simulink model "HybridControllerD2D2"  (R2019a)
settings: Solver=FixedStepDiscrete  StartTime=0.0  StopTime=inf  FixedStep=samplePeriod  RelTol=1e-3  AbsTol=1e-6  EnableMultiTasking=on
PreLoadFcn:
  | initializeSimulation;
  | ATS_setup;
InitFcn:
  | clear('all');
  | initializeSimulation;
  | ATS_setup;
values from neighbouring files (symbols this model uses):
  damperA = 0    [initializeSimulation.m]
  damperB = 0    [initializeSimulation.m]
  damperC = 0    [initializeSimulation.m]
  damperCanon = 1    [initializeSimulation.m]
  flowCanon = 3.85    [initializeSimulation.m]
  forceCanon = 1    [initializeSimulation.m]
  frictionA = 0    [initializeSimulation.m]
  frictionB = 0    [initializeSimulation.m]
  frictionC = 0    [initializeSimulation.m]
  gasConstant = 1.8    [initializeSimulation.m]
  lengthCanon = 1    [initializeSimulation.m]
  massA = 4.2    [initializeSimulation.m]
  massB = 2.5    [initializeSimulation.m]
  massC = 2.5    [initializeSimulation.m]
  massCanon = 0.002588    [initializeSimulation.m]
  maxDisplA = (stroke2A + endLength2A) * lengthCanon    (= 22)    [initializeSimulation.m]
  maxDisplB = (stroke2B + endLength2B) * lengthCanon    (= 42)    [initializeSimulation.m]
  maxDisplC = (stroke2C + endLength2C) * lengthCanon    (= 72)    [initializeSimulation.m]
  maxOilVolume = volume * (1 - (precharge/supplyPress)^(1/gasConstant))    (= 10.5071802963)    [initializeSimulation.m]
  maxVelocA = (maxFlowA * flowCanon / (area1A * areaCanon)) / velocCanon    [initializeSimulation.m]
  maxVelocB = (maxFlowB * flowCanon / (area1B * areaCanon)) / velocCanon    [initializeSimulation.m]
  maxVelocC = (maxFlowC * flowCanon / (area1C * areaCanon)) / velocCanon    [initializeSimulation.m]
  minDisplA = -(stroke1A + endLength1A) * lengthCanon    (= -22)    [initializeSimulation.m]
  minDisplB = -(stroke1B + endLength1B) * lengthCanon    (= -42)    [initializeSimulation.m]
  minDisplC = -(stroke1C + endLength1C) * lengthCanon    (= -72)    [initializeSimulation.m]
  minVelocA = -(maxFlowA * flowCanon / (area2A * areaCanon)) / velocCanon    [initializeSimulation.m]
  minVelocB = -(maxFlowB * flowCanon / (area2B * areaCanon)) / velocCanon    [initializeSimulation.m]
  minVelocC = -(maxFlowC * flowCanon / (area2C * areaCanon)) / velocCanon    [initializeSimulation.m]
  MRC = [2 0.05 0.001]    [ATS_setup.m]
  nAct = 8    [initializeSimulation.m]
  nAdcU = 12    [initializeSimulation.m]
  nDinp = 4    [initializeSimulation.m]
  nDout = 4    [initializeSimulation.m]
  nDucU = 8    [initializeSimulation.m]
  nEncU = 2    [initializeSimulation.m]
  Nl = floor(tl*sample_rate)    [ATS_setup.m]
  P_range = [0.7 1.30 ... (first row only)    [ATS_setup.m]
  precharge = 1000    [initializeSimulation.m]
  pumpFlow = 1e10    (= 10000000000)    [initializeSimulation.m]
  returnPress = 50    [initializeSimulation.m]
  SN = 16    [ATS_setup.m]
  staticForceA = 0    [initializeSimulation.m]
  staticForceB = 0    [initializeSimulation.m]
  staticForceC = 0    [initializeSimulation.m]
  supplyPress = 3000    [initializeSimulation.m]
  velocCanon = 1    [initializeSimulation.m]
  volume = accumVolume * accumNumber    (= 23)    [initializeSimulation.m]
  volumeCanon = 231    [initializeSimulation.m]
  yieldDisplA = 0.1    [initializeSimulation.m]
  yieldDisplB = 0.1    [initializeSimulation.m]
  yieldDisplC = 0.1    [initializeSimulation.m]
  Zden = ztag.Denominator{1}    [ATS_setup.m]
  Znum = ztag.Numerator{1}    [ATS_setup.m]
undefined symbols (not defined in the file or in its folder): DiscIntNeverNeededParam, HybridCtrlParameters, Par, Threshold
libraries: simulink x13
(part 1 of 3)
settings Model: ExtModeTrigMode=oneshot  ExtModeArmWhenConnect=off  ExtModeAutoUpdateStatusClock=off  Creator=Andreas Schellenberg  LastModifiedBy=Andreas
settings SolverCC: AutoScaleAbsTol=off
settings DataIOCC: SaveFormat=Array  SaveOutput=off  SaveTime=off  ReturnWorkspaceOutputs=off  SignalLoggingName=sigsOut
settings OptimizationCC: ExpressionDepthLimit=2147483647  InitFltsAndDblsToZero=on  LifeSpan=inf
settings DebuggingCC: SaveWithParameterizedLinksMsg=none  CheckSSInitialOutputMsg=off  UnderspecifiedInitializationDetection=Classic  MergeDetectMultiDrivingBlocksExec=none  MultiTaskDSMMsg=warning  MultiTaskCondExecSysMsg=none  AllowSymbolicDim=off  StateNameClashWarn=warning  SFUnexpectedBacktrackingDiag=warning  SFNoUnconditionalDefaultTransitionDiag=warning  SFExecutionAtInitializationDiag=none  ArithmeticOperatorsInVariantConditions=warning
settings HardwareCC: ProdBitPerPointer=32  ProdBitPerSizeT=32  ProdBitPerPtrDiffT=32  ProdLargestAtomicFloat=None  ProdIntDivRoundTo=Undefined  ProdEndianess=Unspecified  ProdWordSize=32  ProdHWDeviceType=32-bit Generic  TargetUnknown=on
settings ModelReferenceCC: PropagateSignalLabelsOutOfModel=off
settings SFSimCC: SimCustomHeaderCode="#include \"PredictorCorrector.h\""  SimUserSources=PredictorCorrector.c  SimUseLocalCustomCode=off  SimParseCustomCode=off
settings RTWCC: Description=Generic Real-Time Target  RTWUseLocalCustomCode=off
settings CodeAppCC: StateflowObjectComments=on
settings GRTTargetCC: TargetFcnLib=ansi_tfl_tmw.mat  TargetLangStandard=C89/C90 (ANSI)  GeneratePreprocessorConditionals=Disable all  CombineOutputUpdateFcns=off  GRTInterface=on
settings ConfigComp: CovMetricSettings=dw  CovHtmlReporting=on  CovSaveCumulativeToWorkspaceVar=on  CovSaveSingleToWorkspaceVar=on  CovExternalEMLEnable=off  CovSFcnEnable=off

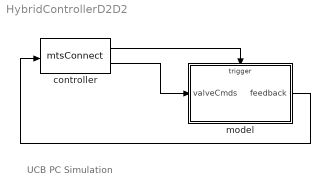
== system HybridControllerD2D2 ==
  note: UCB PC Simulation
  controller : S-Function  FunctionName=mtsConnect  Parameters='127.0.0.1',5002,nUDPInp,nUDPOut  SFunctionDeploymentMode=off  EnableBusSupport=off
  model : Subsystem  TreatAsAtomicUnit=on
  wires:
  model/1(feedback) -> controller/1
  controller/2 -> model/1(valveCmds)
  controller/1 -> model/Trigger

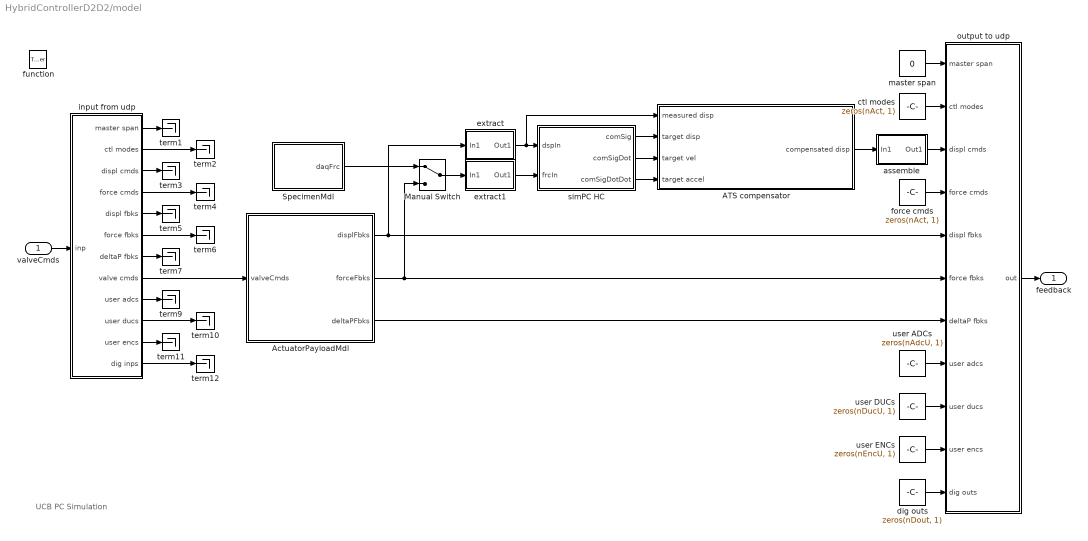
== system HybridControllerD2D2/model ==
  note: UCB PC Simulation
  valveCmds : Inport
  function : TriggerPort  TriggerType=function-call  VariantControl=(inherit)
  ATS compensator : Subsystem  mask(ATS Compensator){param=Par, threshold=Threshold}
      mask prompts: param "Initial a0, a1, a2 values :"; threshold "Threshold values :"
      mask help:
      | Adaptive Time Series (ATS) Compensator
      | by Yunbyeong Chae, Old Dominion University
      | Ref: Chae, Y., Kazemibidokhti, K., and Ricles, J.M. (2013)
      | “Adaptive time series compensator for delay compensation of servo-hydraulic actuator systems for real-time hybrid simulation”,
      | Earthquake Engineering and Structural Dynamics, 42(11), 1697-1715.
  ActuatorPayloadMdl : Subsystem
  Manual Switch : ManualSwitch
  SpecimenMdl : Subsystem
      mask Display: fprintf('Test\nSpecimen');
  assemble : Subsystem  mask(to Actuators){id=1, size=nAct}
      mask prompts: id "Index Vector: id"; size "Vector Size: size"
      mask help: To select to which actuator(s) the signals are going to
      mask Display: disp('Assemble')
  ctl modes : Constant  Value=zeros(nAct, 1)
  dig outs : Constant  Value=zeros(nDout, 1)  OutDataTypeStr=uint32
  extract : Subsystem  mask(from Actuators){id=1, size=nAct}
      mask prompts: id "Index Vector: id"; size "Vector Size: size"
      mask help: To select from which actuator(s) the signals are coming from
      mask Display: disp('Extract')
  extract1 : Subsystem  mask(from Actuators){id=1, size=nAct}
      mask prompts: id "Index Vector: id"; size "Vector Size: size"
      mask help: To select from which actuator(s) the signals are coming from
      mask Display: disp('Extract')
  force cmds : Constant  Value=zeros(nAct, 1)
  input from udp : Subsystem
  master span : Constant  Value=0
  output to udp : Subsystem
  simPC HC : Subsystem  mask(Hybrid Controller: D2/D2){nDOF=HybridCtrlParameters.nDOF, upFact=HybridCtrlParameters.upFact, dtInt=HybridCtrlParameters.dtInt, dtSim=HybridCtrlParameters.dtSim, dtCon=HybridCtrlParameters.dtCon, N=HybridCtrlParameters.N, iDelay=HybridCtrlParameters.iDelay}
      mask prompts: nDOF "Number of DOF: nDOF"; upFact "Upsample Factor: upFact"; dtInt "Integration time step: dtInt"; dtSim "Simulation time step: dtSim"; dtCon "Controller time step: dtCon"; N "Number of substeps: N"; iDelay "Number of delay steps: iDelay"
      mask help: Hybrid Controller using C0-continuous quadratic Lagrange interpolation for prediction and correction
      mask Display: disp('simPC Target\nHybrid Controller\n(D2/D2)')
  term{1..7,9..12} (11 alike) : Terminator
  user ADCs : Constant  Value=zeros(nAdcU, 1)
  user DUCs : Constant  Value=zeros(nDucU, 1)
  user ENCs : Constant  Value=zeros(nEncU, 1)
  feedback : Outport
  wires:
  input from udp/3(displ cmds) -> term3/1
  input from udp/1(master span) -> term1/1
  input from udp/6(force fbks) -> term6/1
  input from udp/10(user ducs) -> term10/1
  input from udp/12(dig inps) -> term12/1
  input from udp/2(ctl modes) -> term2/1
  input from udp/4(force cmds) -> term4/1
  input from udp/5(displ fbks) -> term5/1
  input from udp/7(deltaP fbks) -> term7/1
  input from udp/9(user adcs) -> term9/1
  input from udp/11(user encs) -> term11/1
  valveCmds/1 -> input from udp/1(inp)
  master span/1 -> output to udp/1(master span)
  ctl modes/1 -> output to udp/2(ctl modes)
  assemble/1(Out1) -> output to udp/3(displ cmds)
  force cmds/1 -> output to udp/4(force cmds)
  user ADCs/1 -> output to udp/8(user adcs)
  user DUCs/1 -> output to udp/9(user ducs)
  user ENCs/1 -> output to udp/10(user encs)
  dig outs/1 -> output to udp/11(dig outs)
  output to udp/1(out) -> feedback/1
  ActuatorPayloadMdl/1(displFbks) -> output to udp/5(displ fbks), extract/1(In1)
  ActuatorPayloadMdl/2(forceFbks) -> output to udp/6(force fbks), Manual Switch/2
  ActuatorPayloadMdl/3(deltaPFbks) -> output to udp/7(deltaP fbks)
  input from udp/8(valve cmds) -> ActuatorPayloadMdl/1(valveCmds)
  extract1/1(Out1) -> simPC HC/2(frcIn)
  extract/1(Out1) -> simPC HC/1(dspIn), ATS compensator/1(measured disp)
  simPC HC/2(comSigDot) -> ATS compensator/3(target vel)
  simPC HC/3(comSigDotDot) -> ATS compensator/4(target accel)
  ATS compensator/1(compensated disp) -> assemble/1(In1)
  simPC HC/1(comSig) -> ATS compensator/2(target disp)
  Manual Switch/1 -> extract1/1(In1)
  SpecimenMdl/1(daqFrc) -> Manual Switch/1

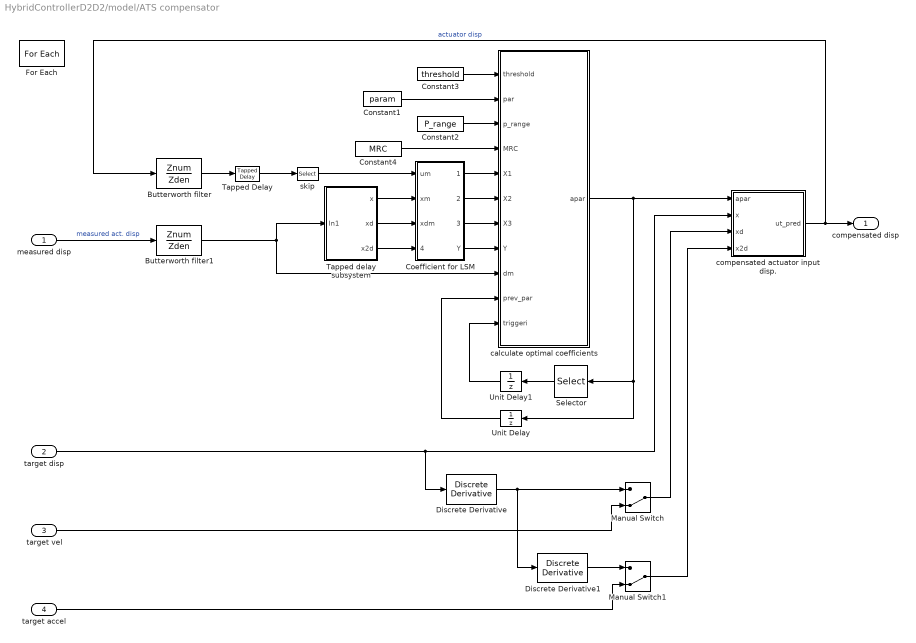
== system HybridControllerD2D2/model/ATS compensator ==
  measured disp : Inport  Partition=on  PartitionDimension=1  PartitionWidth=1  PartitionOffset=0
  target disp : Inport  Port=2  Partition=on  PartitionDimension=1  PartitionWidth=1  PartitionOffset=0
  target vel : Inport  Port=3  Partition=on  PartitionDimension=1  PartitionWidth=1  PartitionOffset=0
  target accel : Inport  Port=4  Partition=on  PartitionDimension=1  PartitionWidth=1  PartitionOffset=0
  Butterworth filter : DiscreteTransferFcn  Numerator=Znum  Denominator=Zden
  Butterworth filter1 : DiscreteTransferFcn  Numerator=Znum  Denominator=Zden
  Coefficient for LSM : Subsystem
  Constant1 : Constant  Value=param
  Constant2 : Constant  Value=P_range
  Constant3 : Constant  Value=threshold
  Constant4 : Constant  Value=MRC
  Discrete Derivative : simulink/Discrete/Discrete Derivative  gainval=1.0  ICPrevScaledInput=0.0  OutMin=[]  OutMax=[]  OutDataType=fixdt(1, 16)  OutScaling=2^-10  DoSatur=off
  Discrete Derivative1 : simulink/Discrete/Discrete Derivative  gainval=1.0  ICPrevScaledInput=0.0  OutMin=[]  OutMax=[]  OutDataType=fixdt(1, 16)  OutScaling=2^-10  DoSatur=off
  For Each : ForEach  DisableCoverage=on  IterateSubsysMaskParameter=on,on  SubsysMaskParameterIterationDimension=2,2  IndexMode=One-based
  Manual Switch : ManualSwitch  CurrentSetting=0
  Manual Switch1 : ManualSwitch  CurrentSetting=0
  Selector : Selector  InputPortWidth=4  IndexOptions=Index vector (dialog)  Indices=4  OutputSizes=1
  Tapped Delay : simulink/Discrete/Tapped Delay  vinit=0.0  samptime=-1  NumDelays=Nl  DelayOrder=Oldest  includeCurrent=off
  Tapped delay subsystem : Subsystem
  Unit Delay : UnitDelay  SampleTime=-1  HasFrameUpgradeWarning=on
  Unit Delay1 : UnitDelay  SampleTime=-1  HasFrameUpgradeWarning=on
  calculate optimal coefficients : MATLAB Function  TreatAsAtomicUnit=on
  compensated actuator input disp. : MATLAB Function  TreatAsAtomicUnit=on
  skip : Selector  InputPortWidth=Nl  IndexOptions=Index vector (dialog)  Indices=[1:SN:Nl]  OutputSizes=1
  compensated disp : Outport  ConcatenationDimension=1
  wires:
  measured disp/1 -> Butterworth filter1/1  "measured act. disp"
  Tapped Delay/1 -> skip/1
  calculate optimal coefficients/1(apar) -> Unit Delay/1, Selector/1, compensated actuator input disp./1(apar)
  compensated actuator input disp./1(ut_pred) -> Butterworth filter/1, compensated disp/1  "actuator disp"
  Constant1/1 -> calculate optimal coefficients/2(par)
  Constant2/1 -> calculate optimal coefficients/3(p_range)
  Unit Delay/1 -> calculate optimal coefficients/10(prev_par)
  target disp/1 -> compensated actuator input disp./2(x), Discrete Derivative/1
  skip/1 -> Coefficient for LSM/1(um)
  Tapped delay subsystem/1(x) -> Coefficient for LSM/2(xm)
  Tapped delay subsystem/2(xd) -> Coefficient for LSM/3(xdm)
  Tapped delay subsystem/3(x2d) -> Coefficient for LSM/4(x2dm)
  Coefficient for LSM/1(X(1,:)) -> calculate optimal coefficients/5(X1)
  Coefficient for LSM/2(X(2,:)) -> calculate optimal coefficients/6(X2)
  Coefficient for LSM/3(X(3,:)) -> calculate optimal coefficients/7(X3)
  Coefficient for LSM/4(Y) -> calculate optimal coefficients/8(Y)
  Unit Delay1/1 -> calculate optimal coefficients/11(triggeri)
  Constant3/1 -> calculate optimal coefficients/1(threshold)
  Butterworth filter/1 -> Tapped Delay/1
  Constant4/1 -> calculate optimal coefficients/4(MRC)
  Selector/1 -> Unit Delay1/1
  Manual Switch/1 -> compensated actuator input disp./3(xd)
  Discrete Derivative/1 -> Manual Switch/1, Discrete Derivative1/1
  target vel/1 -> Manual Switch/2
  Discrete Derivative1/1 -> Manual Switch1/1
  Manual Switch1/1 -> compensated actuator input disp./4(x2d)
  target accel/1 -> Manual Switch1/2
  Butterworth filter1/1 -> Tapped delay subsystem/1(In1), calculate optimal coefficients/9(dm)

== system HybridControllerD2D2/model/ActuatorPayloadMdl ==
  valveCmds : Inport
  Demux : Demux  Outputs=nAct
  Mux : Mux  Inputs=nAct
  Mux1 : Mux  Inputs=nAct
  Mux2 : Mux  Inputs=nAct
  Sum : Sum  Inputs=++++++++  SaturateOnIntegerOverflow=on
  accumulators : Subsystem
  dynamic long channel #1 : Subsystem
  dynamic long channel #2 : Subsystem
  dynamic short channel #1 : Subsystem
  dynamic short channel #2 : Subsystem
  static channel #1 : Subsystem
  static channel #2 : Subsystem
  static channel #3 : Subsystem
  static channel #4 : Subsystem
  displFbks : Outport
  forceFbks : Outport  Port=2
  deltaPFbks : Outport  Port=3
  wires:
  Demux/1 -> dynamic short channel #1/1(valve cmd)
  Demux/3 -> dynamic long channel #1/1(valve cmd)
  Demux/2 -> dynamic short channel #2/1(valve cmd)
  dynamic short channel #1/4(flow) -> Sum/1
  dynamic short channel #2/4(flow) -> Sum/2
  dynamic long channel #1/4(flow) -> Sum/3
  Sum/1 -> accumulators/1(flow)
  Demux/4 -> dynamic long channel #2/1(valve cmd)
  Demux/5 -> static channel #1/1(valve cmd)
  Demux/6 -> static channel #2/1(valve cmd)
  Demux/7 -> static channel #3/1(valve cmd)
  Demux/8 -> static channel #4/1(valve cmd)
  dynamic long channel #2/4(flow) -> Sum/4
  static channel #1/4(flow) -> Sum/5
  static channel #2/4(flow) -> Sum/6
  static channel #3/4(flow) -> Sum/7
  static channel #4/4(flow) -> Sum/8
  accumulators/1(press) -> static channel #4/2(spl press), static channel #3/2(spl press), static channel #2/2(spl press), static channel #1/2(spl press), dynamic long channel #2/2(spl press), dynamic long channel #1/2(spl press), dynamic short channel #2/2(spl press), dynamic short channel #1/2(spl press)
  dynamic short channel #1/1(displ) -> Mux/1
  dynamic short channel #2/1(displ) -> Mux/2
  dynamic long channel #1/1(displ) -> Mux/3
  dynamic long channel #2/1(displ) -> Mux/4
  static channel #1/1(displ) -> Mux/5
  static channel #2/1(displ) -> Mux/6
  static channel #3/1(displ) -> Mux/7
  static channel #4/1(displ) -> Mux/8
  dynamic short channel #1/2(force) -> Mux1/1
  dynamic short channel #2/2(force) -> Mux1/2
  dynamic long channel #1/2(force) -> Mux1/3
  dynamic long channel #2/2(force) -> Mux1/4
  static channel #1/2(force) -> Mux1/5
  static channel #2/2(force) -> Mux1/6
  static channel #3/2(force) -> Mux1/7
  static channel #4/2(force) -> Mux1/8
  dynamic short channel #1/3(dpforce) -> Mux2/1
  dynamic short channel #2/3(dpforce) -> Mux2/2
  dynamic long channel #1/3(dpforce) -> Mux2/3
  dynamic long channel #2/3(dpforce) -> Mux2/4
  static channel #1/3(dpforce) -> Mux2/5
  static channel #2/3(dpforce) -> Mux2/6
  static channel #3/3(dpforce) -> Mux2/7
  static channel #4/3(dpforce) -> Mux2/8
  valveCmds/1 -> Demux/1
  Mux/1 -> displFbks/1
  Mux1/1 -> forceFbks/1
  Mux2/1 -> deltaPFbks/1

== system HybridControllerD2D2/model/SpecimenMdl ==
  Scope3 : Scope
  Specimen #1 : S-Function  FunctionName=SFun_SimFEAdapter  Parameters=ipAddr,ipPort,dataSize  SFunctionDeploymentMode=off  EnableBusSupport=off  mask(SimFEAdapter){ipAddr=127.0.0.1, ipPort=44000, dataSize=256}
      mask prompts: ipAddr "IP Address of Adapter Element"; ipPort "IP Port Number of Adapter Element"; dataSize "Size of Data Arrays"
      mask Display: disp('SimFE\nAdapter');
  Terminator : Terminator
  assemble1 : Subsystem  mask(to Actuators){id=1, size=nAct}
      mask prompts: id "Index Vector: id"; size "Vector Size: size"
      mask help: To select to which actuator(s) the signals are going to
      mask Display: disp('Assemble')
  assemble2 : Subsystem  mask(to Actuators){id=1, size=nAct}
      mask prompts: id "Index Vector: id"; size "Vector Size: size"
      mask help: To select to which actuator(s) the signals are going to
      mask Display: disp('Assemble')
  extract2 : Subsystem  mask(from Actuators){id=1, size=nAct}
      mask prompts: id "Index Vector: id"; size "Vector Size: size"
      mask help: To select from which actuator(s) the signals are coming from
      mask Display: disp('Extract')
  from Actuators : Subsystem
  to LoadCells : Subsystem
  daqFrc : Outport
  wires:
  from Actuators/1(ctrlDisp) -> extract2/1(In1)
  extract2/1(Out1) -> Specimen #1/1
  Specimen #1/1 -> assemble2/1(In1)
  Specimen #1/2 -> assemble1/1(In1), Scope3/1
  assemble2/1(Out1) -> Terminator/1
  assemble1/1(Out1) -> daqFrc/1, to LoadCells/1(daqForce)

== system HybridControllerD2D2/model/assemble ==
  In1 : Inport
  Assignment : Assignment  OutputInitialize=Specify size for each dimension in table  IndexOptions=Index vector (port)  Indices=1  OutputSizes=nAct
  Constant : Constant  Value=id
  Out1 : Outport
  wires:
  Constant/1 -> Assignment/2
  Assignment/1 -> Out1/1
  In1/1 -> Assignment/1

== system HybridControllerD2D2/model/extract ==
  In1 : Inport
  Selector : Selector  InputPortWidth=size  IndexOptions=Index vector (dialog)  Indices=id  OutputSizes=1
  Out1 : Outport
  wires:
  Selector/1 -> Out1/1
  In1/1 -> Selector/1

== system HybridControllerD2D2/model/extract1 ==
  In1 : Inport
  Selector : Selector  InputPortWidth=size  IndexOptions=Index vector (dialog)  Indices=id  OutputSizes=1
  Out1 : Outport
  wires:
  Selector/1 -> Out1/1
  In1/1 -> Selector/1

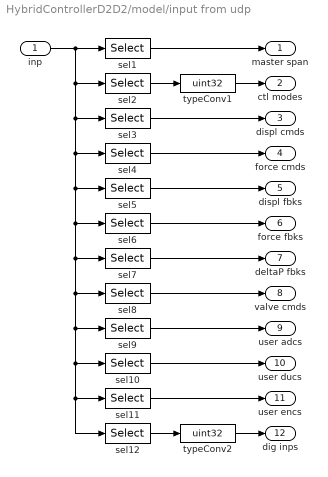
== system HybridControllerD2D2/model/input from udp ==
  inp : Inport
  sel1 : Selector  InputPortWidth=nUDPOut  IndexOptions=Index vector (dialog)  Indices=[0]+1  OutputSizes=1
  sel10 : Selector  InputPortWidth=nUDPOut  IndexOptions=Index vector (dialog)  Indices=[1:nDucU]+1+7*nAct+nAdcU  OutputSizes=1
  sel11 : Selector  InputPortWidth=nUDPOut  IndexOptions=Index vector (dialog)  Indices=[1:nEncU]+1+7*nAct+nAdcU+nDucU  OutputSizes=1
  sel12 : Selector  InputPortWidth=nUDPOut  IndexOptions=Index vector (dialog)  Indices=[1:nDinp]+1+7*nAct+nAdcU+nDucU+nEncU  OutputSizes=1
  sel2 : Selector  InputPortWidth=nUDPOut  IndexOptions=Index vector (dialog)  Indices=[1:nAct]+1+0*nAct  OutputSizes=1
  sel3 : Selector  InputPortWidth=nUDPOut  IndexOptions=Index vector (dialog)  Indices=[1:nAct]+1+1*nAct  OutputSizes=1
  sel4 : Selector  InputPortWidth=nUDPOut  IndexOptions=Index vector (dialog)  Indices=[1:nAct]+1+2*nAct  OutputSizes=1
  sel5 : Selector  InputPortWidth=nUDPOut  IndexOptions=Index vector (dialog)  Indices=[1:nAct]+1+3*nAct  OutputSizes=1
  sel6 : Selector  InputPortWidth=nUDPOut  IndexOptions=Index vector (dialog)  Indices=[1:nAct]+1+4*nAct  OutputSizes=1
  sel7 : Selector  InputPortWidth=nUDPOut  IndexOptions=Index vector (dialog)  Indices=[1:nAct]+1+5*nAct  OutputSizes=1
  sel8 : Selector  InputPortWidth=nUDPOut  IndexOptions=Index vector (dialog)  Indices=[1:nAct]+1+6*nAct  OutputSizes=1
  sel9 : Selector  InputPortWidth=nUDPOut  IndexOptions=Index vector (dialog)  Indices=[1:nAdcU]+1+7*nAct  OutputSizes=1
  typeConv1 : DataTypeConversion  OutDataTypeStr=uint32  SaturateOnIntegerOverflow=on  RndMeth=Zero
  typeConv2 : DataTypeConversion  OutDataTypeStr=uint32  SaturateOnIntegerOverflow=on  RndMeth=Zero
  master span : Outport
  ctl modes : Outport  Port=2
  displ cmds : Outport  Port=3
  force cmds : Outport  Port=4
  displ fbks : Outport  Port=5
  force fbks : Outport  Port=6
  deltaP fbks : Outport  Port=7
  valve cmds : Outport  Port=8
  user adcs : Outport  Port=9
  user ducs : Outport  Port=10
  user encs : Outport  Port=11
  dig inps : Outport  Port=12
  wires:
  sel1/1 -> master span/1
  sel2/1 -> typeConv1/1
  sel3/1 -> displ cmds/1
  sel4/1 -> force cmds/1
  sel5/1 -> displ fbks/1
  sel6/1 -> force fbks/1
  sel7/1 -> deltaP fbks/1
  sel8/1 -> valve cmds/1
  sel9/1 -> user adcs/1
  sel10/1 -> user ducs/1
  sel11/1 -> user encs/1
  sel12/1 -> typeConv2/1
  inp/1 -> sel1/1, sel2/1, sel3/1, sel11/1, sel12/1, sel10/1, sel9/1, sel8/1, sel7/1, sel6/1, sel5/1, sel4/1
  typeConv1/1 -> ctl modes/1
  typeConv2/1 -> dig inps/1

== system HybridControllerD2D2/model/output to udp ==
  master span : Inport
  ctl modes : Inport  Port=2
  displ cmds : Inport  Port=3
  force cmds : Inport  Port=4
  displ fbks : Inport  Port=5
  force fbks : Inport  Port=6
  deltaP fbks : Inport  Port=7
  user adcs : Inport  Port=8
  user ducs : Inport  Port=9
  user encs : Inport  Port=10
  dig outs : Inport  Port=11
  Mux : Mux  Inputs=11
  typeConv1 : DataTypeConversion  OutDataTypeStr=double  SaturateOnIntegerOverflow=on  RndMeth=Zero
  typeConv2 : DataTypeConversion  OutDataTypeStr=double  SaturateOnIntegerOverflow=on  RndMeth=Zero
  out : Outport
  wires:
  typeConv2/1 -> Mux/11
  dig outs/1 -> typeConv2/1
  user encs/1 -> Mux/10
  user ducs/1 -> Mux/9
  user adcs/1 -> Mux/8
  deltaP fbks/1 -> Mux/7
  force fbks/1 -> Mux/6
  displ fbks/1 -> Mux/5
  force cmds/1 -> Mux/4
  master span/1 -> Mux/1
  displ cmds/1 -> Mux/3
  ctl modes/1 -> typeConv1/1
  Mux/1 -> out/1
  typeConv1/1 -> Mux/2

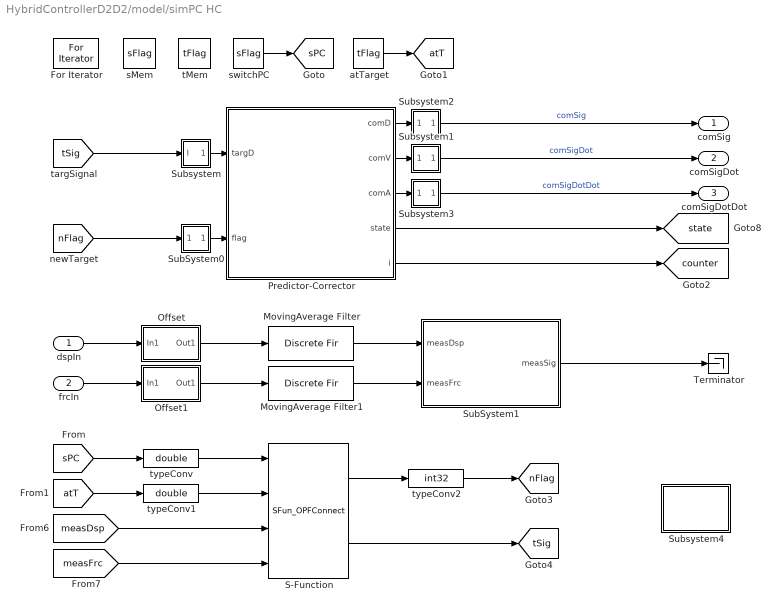
== system HybridControllerD2D2/model/simPC HC ==
  dspIn : Inport
  frcIn : Inport  Port=2
  For Iterator : ForIterator  IterationLimit=upFact  ShowIterationPort=off
  MovingAverage Filter : DiscreteFir  Coefficients=1/numSample*ones(1,numSample)  mask(Moving Average Filter){numSample=1}
      mask prompts: numSample "Number of Samples: numSample"
      mask help:
      | Moving average filter by using discrete FIR filter.
      | Set numSample = 1 for no filtering.
      mask Display: fprintf('MovingAverage\nFilter')
  MovingAverage Filter1 : DiscreteFir  Coefficients=1/numSample*ones(1,numSample)  mask(Moving Average Filter){numSample=1}
      mask prompts: numSample "Number of Samples: numSample"
      mask help:
      | Moving average filter by using discrete FIR filter.
      | Set numSample = 1 for no filtering.
      mask Display: fprintf('MovingAverage\nFilter')
  Offset : Subsystem  mask(Signal Offset){nS=nDOF, nOffset=-1}
      mask prompts: nS "Number of Signals: nS"; nOffset "Number of samples to initialize offset: nOffset"
      mask help:
      | Offset signal by average of signal over initial number of samples.
      | Set nOffset = -1 for no signal offset.
      mask Display: fprintf('Signal\nOffset')
  Offset1 : Subsystem  mask(Signal Offset){nS=nDOF, nOffset=-1}
      mask prompts: nS "Number of Signals: nS"; nOffset "Number of samples to initialize offset: nOffset"
      mask help:
      | Offset signal by average of signal over initial number of samples.
      | Set nOffset = -1 for no signal offset.
      mask Display: fprintf('Signal\nOffset')
  Predictor-Corrector : Stateflow chart  TreatAsAtomicUnit=on
  S-Function : S-Function  FunctionName=SFun_OPFConnect  Parameters=ipPort  SFunctionDeploymentMode=off  EnableBusSupport=off  mask(OpenFresco Connect){ipPort=8090}
      mask prompts: ipPort "IP Port Number of Server"
      mask Display: disp('OpenFresco\nConnect');
  SubSystem0 : Subsystem
      mask Display: disp('I/O')
  SubSystem1 : Subsystem
  Subsystem : Subsystem
      mask Display: disp('I/O')
  Subsystem1 : Subsystem
      mask Display: disp('I/O')
  Subsystem2 : Subsystem
      mask Display: disp('I/O')
  Subsystem3 : Subsystem
      mask Display: disp('I/O')
  Subsystem4 : Subsystem
      mask Display: disp('Scopes')
  Terminator : Terminator
  atTarget : DataStoreRead  DataStoreName=tFlag
  sMem : DataStoreMemory  DataStoreName=sFlag  ShowAdditionalParam=off  OutDataTypeStr=int32
  switchPC : DataStoreRead  DataStoreName=sFlag
  tMem : DataStoreMemory  DataStoreName=tFlag  ShowAdditionalParam=off  OutDataTypeStr=int32
  typeConv : DataTypeConversion  OutDataTypeStr=double  RndMeth=Round  SaturateOnIntegerOverflow=on
  typeConv1 : DataTypeConversion  OutDataTypeStr=double  RndMeth=Round  SaturateOnIntegerOverflow=on
  typeConv2 : DataTypeConversion  OutDataTypeStr=int32  RndMeth=Round  SaturateOnIntegerOverflow=on
  comSig : Outport
  comSigDot : Outport  Port=2
  comSigDotDot : Outport  Port=3
  tag scope: atT=global, counter=global, nFlag=global, sPC=global, state=global, tSig=global
  wires:
  SubSystem0/1(Out) -> Predictor-Corrector/2(flag)
  [nFlag] -> SubSystem0/1(In)
  [tSig] -> Subsystem/1(I)
  [sPC] -> typeConv/1
  [atT] -> typeConv1/1
  S-Function/1 -> typeConv2/1
  S-Function/2 -> [tSig]
  Subsystem/1(O) -> Predictor-Corrector/1(targD)
  Subsystem2/1(Out) -> comSig/1  "comSig"
  switchPC/1 -> [sPC]
  atTarget/1 -> [atT]
  Predictor-Corrector/1(comD) -> Subsystem2/1(In)
  Subsystem1/1(Out) -> comSigDot/1  "comSigDot"
  Predictor-Corrector/2(comV) -> Subsystem1/1(In)
  Subsystem3/1(Out) -> comSigDotDot/1  "comSigDotDot"
  Predictor-Corrector/3(comA) -> Subsystem3/1(In)
  frcIn/1 -> Offset1/1(In1)
  SubSystem1/1(measSig) -> Terminator/1
  dspIn/1 -> Offset/1(In1)
  MovingAverage Filter/1 -> SubSystem1/1(measDsp)
  MovingAverage Filter1/1 -> SubSystem1/2(measFrc)
  Offset/1(Out1) -> MovingAverage Filter/1
  Offset1/1(Out1) -> MovingAverage Filter1/1
  Predictor-Corrector/5(i) -> [counter]
  Predictor-Corrector/4(state) -> [state]
  [measFrc] -> S-Function/4
  [measDsp] -> S-Function/3
  typeConv/1 -> S-Function/1
  typeConv1/1 -> S-Function/2
  typeConv2/1 -> [nFlag]

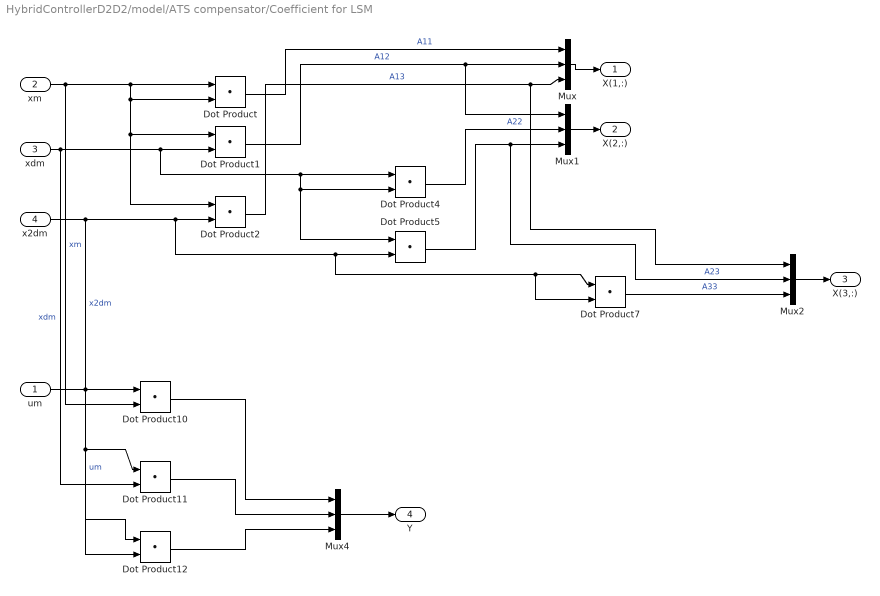
== system HybridControllerD2D2/model/ATS compensator/Coefficient for LSM ==
  um : Inport
  xm : Inport  Port=2
  xdm : Inport  Port=3
  x2dm : Inport  Port=4
  Dot Product{,1..2,4..5,7,10..12} (9 alike) : DotProduct  InputSameDT=on  OutDataTypeStr=Inherit: Inherit via internal rule
  Mux{,1..2,4} (4 alike) : Mux  Inputs=3
  X(1,:) : Outport
  X(2,:) : Outport  Port=2
  X(3,:) : Outport  Port=3
  Y : Outport  Port=4
  wires:
  xm/1 -> Dot Product/1, Dot Product/2, Dot Product1/1, Dot Product2/1, Dot Product10/2  "xm"
  xdm/1 -> Dot Product1/2, Dot Product4/1, Dot Product4/2, Dot Product5/1, Dot Product11/2  "xdm"
  x2dm/1 -> Dot Product2/2, Dot Product5/2, Dot Product7/1, Dot Product7/2, Dot Product12/2  "x2dm"
  um/1 -> Dot Product10/1, Dot Product11/1, Dot Product12/1  "um"
  Dot Product/1 -> Mux/1  "A11"
  Dot Product1/1 -> Mux/2, Mux1/1  "A12"
  Dot Product2/1 -> Mux/3, Mux2/1  "A13"
  Mux/1 -> X(1,:)/1
  Dot Product4/1 -> Mux1/2  "A22"
  Dot Product5/1 -> Mux1/3, Mux2/2  "A23"
  Mux1/1 -> X(2,:)/1
  Dot Product7/1 -> Mux2/3  "A33"
  Mux2/1 -> X(3,:)/1
  Mux4/1 -> Y/1
  Dot Product10/1 -> Mux4/1
  Dot Product11/1 -> Mux4/2
  Dot Product12/1 -> Mux4/3

== system HybridControllerD2D2/model/ATS compensator/Tapped delay subsystem ==
  In1 : Inport
  Discrete Derivative : simulink/Discrete/Discrete Derivative  gainval=1.0  ICPrevScaledInput=0.0  OutMin=[]  OutMax=[]  OutDataType=fixdt(1, 16)  OutScaling=2^-10  DoSatur=off
  Discrete Derivative1 : simulink/Discrete/Discrete Derivative  gainval=1.0  ICPrevScaledInput=0.0  OutMin=[]  OutMax=[]  OutDataType=fixdt(1, 16)  OutScaling=2^-10  DoSatur=off
  Tapped Delay : simulink/Discrete/Tapped Delay  vinit=0.0  samptime=-1  NumDelays=Nl  DelayOrder=Oldest  includeCurrent=off
  Tapped Delay1 : simulink/Discrete/Tapped Delay  vinit=0.0  samptime=-1  NumDelays=Nl  DelayOrder=Oldest  includeCurrent=off
  Tapped Delay2 : simulink/Discrete/Tapped Delay  vinit=0.0  samptime=-1  NumDelays=Nl  DelayOrder=Oldest  includeCurrent=off
  skip : Selector  InputPortWidth=Nl  IndexOptions=Index vector (dialog)  Indices=[1:SN:Nl]  OutputSizes=1
  skip1 : Selector  InputPortWidth=Nl  IndexOptions=Index vector (dialog)  Indices=[1:SN:Nl]  OutputSizes=1
  skip2 : Selector  InputPortWidth=Nl  IndexOptions=Index vector (dialog)  Indices=[1:SN:Nl]  OutputSizes=1
  x : Outport
  xd : Outport  Port=2
  x2d : Outport  Port=3
  wires:
  In1/1 -> Discrete Derivative/1, Tapped Delay/1
  Discrete Derivative/1 -> Discrete Derivative1/1, Tapped Delay1/1
  Discrete Derivative1/1 -> Tapped Delay2/1
  Tapped Delay/1 -> skip/1
  Tapped Delay1/1 -> skip1/1
  Tapped Delay2/1 -> skip2/1
  skip/1 -> x/1
  skip1/1 -> xd/1
  skip2/1 -> x2d/1

== system HybridControllerD2D2/model/ActuatorPayloadMdl/accumulators ==
  flow : Inport
  Sum : Sum  Inputs=+-|  SaturateOnIntegerOverflow=on  InputSameDT=on  OutDataTypeStr=Inherit: Same as first input
  Sum1 : Sum  Inputs=+-|  SaturateOnIntegerOverflow=on  InputSameDT=on  OutDataTypeStr=Inherit: Same as first input
  bottle volume : Constant  Value=volume*volumeCanon
  flowCanon : Gain  Gain=flowCanon  SaturateOnIntegerOverflow=on  OutDataTypeStr=Inherit: Same as input  ParamDataTypeStr=Inherit: Same as input
  gas constant : Constant  Value=gasConstant
  initial condition : UnitDelay  InitialCondition=supplyPress  SampleTime=-1  HasFrameUpgradeWarning=on
  integrator : DiscreteIntegrator  InitialCondition=maxOilVolume*volumeCanon  SampleTime=-1  LimitOutput=on  UpperSaturationLimit=maxOilVolume*volumeCanon  LowerSaturationLimit=0  ICPrevOutput=DiscIntNeverNeededParam  ICPrevScaledInput=DiscIntNeverNeededParam
  power : Math  Operator=pow  SaturateOnIntegerOverflow=on
  precharge : Gain  Gain=precharge  SaturateOnIntegerOverflow=on  OutDataTypeStr=Inherit: Same as input  ParamDataTypeStr=Inherit: Same as input
  pump flow : Constant  Value=pumpFlow
  quotient : Product  Inputs=*/  SaturateOnIntegerOverflow=on  InputSameDT=on  OutDataTypeStr=Inherit: Same as first input
  press : Outport
  wires:
  initial condition/1 -> press/1
  flowCanon/1 -> integrator/1
  flow/1 -> Sum/2
  integrator/1 -> Sum1/2  "current oil volume"
  quotient/1 -> power/1
  Sum1/1 -> quotient/2  "current gas volume"
  precharge/1 -> initial condition/1
  power/1 -> precharge/1
  gas constant/1 -> power/2
  bottle volume/1 -> quotient/1, Sum1/1
  Sum/1 -> flowCanon/1
  pump flow/1 -> Sum/1

== system HybridControllerD2D2/model/ActuatorPayloadMdl/dynamic long channel #1 ==
  valve cmd : Inport
  spl press : Inport  Port=2
  actuator/valve model : Subsystem  mask(Inverse Actuator){}
  payload : Subsystem
  return pressure : Constant  Value=returnPress
  displ : Outport
  force : Outport  Port=2
  dpforce : Outport  Port=3
  flow : Outport  Port=4
  wires:
  payload/2(veloc) -> actuator/valve model/3(veloc)
  payload/1(displ) -> displ/1, actuator/valve model/2(displ)
  valve cmd/1 -> actuator/valve model/1(cmd)
  return pressure/1 -> actuator/valve model/5(rtn press)
  spl press/1 -> actuator/valve model/4(spl press)
  actuator/valve model/2(flow) -> flow/1
  actuator/valve model/1(force) -> force/1, dpforce/1, payload/1(force)

== system HybridControllerD2D2/model/ActuatorPayloadMdl/dynamic long channel #2 ==
  valve cmd : Inport
  spl press : Inport  Port=2
  actuator/valve model : Subsystem  mask(Inverse Actuator){}
  payload : Subsystem
  return pressure : Constant  Value=returnPress
  displ : Outport
  force : Outport  Port=2
  dpforce : Outport  Port=3
  flow : Outport  Port=4
  wires:
  actuator/valve model/1(force) -> dpforce/1, force/1, payload/1(force)
  actuator/valve model/2(flow) -> flow/1
  spl press/1 -> actuator/valve model/4(spl press)
  return pressure/1 -> actuator/valve model/5(rtn press)
  valve cmd/1 -> actuator/valve model/1(cmd)
  payload/1(displ) -> actuator/valve model/2(displ), displ/1
  payload/2(veloc) -> actuator/valve model/3(veloc)

== system HybridControllerD2D2/model/ActuatorPayloadMdl/dynamic short channel #1 ==
  valve cmd : Inport
  spl press : Inport  Port=2
  actuator/valve model : Subsystem  mask(Inverse Actuator){}
  payload : Subsystem
  return pressure : Constant  Value=returnPress
  displ : Outport
  force : Outport  Port=2
  dpforce : Outport  Port=3
  flow : Outport  Port=4
  wires:
  actuator/valve model/1(force) -> dpforce/1, force/1, payload/1(force)
  actuator/valve model/2(flow) -> flow/1
  spl press/1 -> actuator/valve model/4(spl press)
  return pressure/1 -> actuator/valve model/5(rtn press)
  valve cmd/1 -> actuator/valve model/1(cmd)
  payload/1(displ) -> actuator/valve model/2(displ), displ/1
  payload/2(veloc) -> actuator/valve model/3(veloc)

== system HybridControllerD2D2/model/ActuatorPayloadMdl/dynamic short channel #2 ==
  valve cmd : Inport
  spl press : Inport  Port=2
  actuator/valve model : Subsystem  mask(Inverse Actuator){}
  payload : Subsystem
  return pressure : Constant  Value=returnPress
  displ : Outport
  force : Outport  Port=2
  dpforce : Outport  Port=3
  flow : Outport  Port=4
  wires:
  actuator/valve model/1(force) -> dpforce/1, force/1, payload/1(force)
  actuator/valve model/2(flow) -> flow/1
  spl press/1 -> actuator/valve model/4(spl press)
  return pressure/1 -> actuator/valve model/5(rtn press)
  valve cmd/1 -> actuator/valve model/1(cmd)
  payload/1(displ) -> actuator/valve model/2(displ), displ/1
  payload/2(veloc) -> actuator/valve model/3(veloc)

== system HybridControllerD2D2/model/ActuatorPayloadMdl/static channel #1 ==
  valve cmd : Inport
  spl press : Inport  Port=2
  actuator/valve model : Subsystem  mask(Inverse Actuator){}
  payload : Subsystem
  return pressure : Constant  Value=returnPress
  displ : Outport
  force : Outport  Port=2
  dpforce : Outport  Port=3
  flow : Outport  Port=4
  wires:
  payload/2(veloc) -> actuator/valve model/3(veloc)
  payload/1(displ) -> displ/1, actuator/valve model/2(displ)
  valve cmd/1 -> actuator/valve model/1(cmd)
  return pressure/1 -> actuator/valve model/5(rtn press)
  spl press/1 -> actuator/valve model/4(spl press)
  actuator/valve model/2(flow) -> flow/1
  actuator/valve model/1(force) -> force/1, dpforce/1, payload/1(force)

== system HybridControllerD2D2/model/ActuatorPayloadMdl/static channel #2 ==
  valve cmd : Inport
  spl press : Inport  Port=2
  actuator/valve model : Subsystem  mask(Inverse Actuator){}
  payload : Subsystem
  return pressure : Constant  Value=returnPress
  displ : Outport
  force : Outport  Port=2
  dpforce : Outport  Port=3
  flow : Outport  Port=4
  wires:
  actuator/valve model/1(force) -> dpforce/1, force/1, payload/1(force)
  actuator/valve model/2(flow) -> flow/1
  spl press/1 -> actuator/valve model/4(spl press)
  return pressure/1 -> actuator/valve model/5(rtn press)
  valve cmd/1 -> actuator/valve model/1(cmd)
  payload/1(displ) -> actuator/valve model/2(displ), displ/1
  payload/2(veloc) -> actuator/valve model/3(veloc)

== system HybridControllerD2D2/model/ActuatorPayloadMdl/static channel #3 ==
  valve cmd : Inport
  spl press : Inport  Port=2
  actuator/valve model : Subsystem  mask(Inverse Actuator){}
  payload : Subsystem
  return pressure : Constant  Value=returnPress
  displ : Outport
  force : Outport  Port=2
  dpforce : Outport  Port=3
  flow : Outport  Port=4
  wires:
  payload/2(veloc) -> actuator/valve model/3(veloc)
  payload/1(displ) -> displ/1, actuator/valve model/2(displ)
  valve cmd/1 -> actuator/valve model/1(cmd)
  return pressure/1 -> actuator/valve model/5(rtn press)
  spl press/1 -> actuator/valve model/4(spl press)
  actuator/valve model/2(flow) -> flow/1
  actuator/valve model/1(force) -> force/1, dpforce/1, payload/1(force)

== system HybridControllerD2D2/model/ActuatorPayloadMdl/static channel #4 ==
  valve cmd : Inport
  spl press : Inport  Port=2
  actuator/valve model : Subsystem  mask(Inverse Actuator){}
  payload : Subsystem
  return pressure : Constant  Value=returnPress
  displ : Outport
  force : Outport  Port=2
  dpforce : Outport  Port=3
  flow : Outport  Port=4
  wires:
  actuator/valve model/1(force) -> dpforce/1, force/1, payload/1(force)
  actuator/valve model/2(flow) -> flow/1
  spl press/1 -> actuator/valve model/4(spl press)
  return pressure/1 -> actuator/valve model/5(rtn press)
  valve cmd/1 -> actuator/valve model/1(cmd)
  payload/1(displ) -> actuator/valve model/2(displ), displ/1
  payload/2(veloc) -> actuator/valve model/3(veloc)

== system HybridControllerD2D2/model/SpecimenMdl/assemble1 ==
  In1 : Inport
  Assignment : Assignment  OutputInitialize=Specify size for each dimension in table  IndexOptions=Index vector (port)  Indices=1  OutputSizes=nAct
  Constant : Constant  Value=id
  Out1 : Outport
  wires:
  Constant/1 -> Assignment/2
  Assignment/1 -> Out1/1
  In1/1 -> Assignment/1

== system HybridControllerD2D2/model/SpecimenMdl/assemble2 ==
  In1 : Inport
  Assignment : Assignment  OutputInitialize=Specify size for each dimension in table  IndexOptions=Index vector (port)  Indices=1  OutputSizes=nAct
  Constant : Constant  Value=id
  Out1 : Outport
  wires:
  Constant/1 -> Assignment/2
  Assignment/1 -> Out1/1
  In1/1 -> Assignment/1

== system HybridControllerD2D2/model/SpecimenMdl/extract2 ==
  In1 : Inport
  Selector : Selector  InputPortWidth=size  IndexOptions=Index vector (dialog)  Indices=id  OutputSizes=1
  Out1 : Outport
  wires:
  Selector/1 -> Out1/1
  In1/1 -> Selector/1

== system HybridControllerD2D2/model/SpecimenMdl/from Actuators ==
  Bus Creator : BusCreator  Inputs=8
  ctrlDisp : Outport
  wires:
  [ch1a] -> Bus Creator/1
  [ch2a] -> Bus Creator/2
  [ch3a] -> Bus Creator/3
  [ch4a] -> Bus Creator/4
  [ch5a] -> Bus Creator/5
  [ch6a] -> Bus Creator/6
  [ch7a] -> Bus Creator/7
  [ch8a] -> Bus Creator/8
  Bus Creator/1 -> ctrlDisp/1

== system HybridControllerD2D2/model/SpecimenMdl/to LoadCells ==
  daqForce : Inport
  Demux : Demux  Outputs=8
  tag scope: ch1b=global, ch2b=global, ch3b=global, ch4b=global, ch5b=global, ch6b=global, ch7b=global, ch8b=global
  wires:
  Demux/1 -> [ch1b]
  Demux/2 -> [ch2b]
  Demux/3 -> [ch3b]
  Demux/4 -> [ch4b]
  Demux/5 -> [ch5b]
  Demux/6 -> [ch6b]
  Demux/7 -> [ch7b]
  Demux/8 -> [ch8b]
  daqForce/1 -> Demux/1

== system HybridControllerD2D2/model/simPC HC/Offset ==
  In1 : Inport
  Constant : Constant  Value=zeros(1,nS)
  Counter : simulink/Sources/Counter Free-Running  NumBits=32  tsamp=-1
  Data Store Memory : DataStoreMemory  DataStoreName=x0  InitialValue=zeros(1,nS)  ShowAdditionalParam=off  OutDataTypeStr=double
  Data Store Read : DataStoreRead  DataStoreName=x0
  If : If  IfExpression=u1 < nOffset  ShowElse=off
  If Action : Subsystem  TreatAsAtomicUnit=on
  Sum1 : Sum  Inputs=+-|  SaturateOnIntegerOverflow=on  InputSameDT=on  OutDataTypeStr=Inherit: Same as first input
  Switch : Switch  Threshold=nOffset  SaturateOnIntegerOverflow=on  InputSameDT=on
  typeConv : DataTypeConversion  OutDataTypeStr=double  RndMeth=Round  SaturateOnIntegerOverflow=on
  Out1 : Outport
  wires:
  Switch/1 -> Out1/1
  Sum1/1 -> Switch/1
  Data Store Read/1 -> Sum1/2
  In1/1 -> If Action/1(In1), Sum1/1
  Constant/1 -> Switch/3
  Counter/1 -> typeConv/1
  If/1 -> If Action/Action
  typeConv/1 -> Switch/2, If/1

== system HybridControllerD2D2/model/simPC HC/Offset1 ==
  In1 : Inport
  Constant : Constant  Value=zeros(1,nS)
  Counter : simulink/Sources/Counter Free-Running  NumBits=32  tsamp=-1
  Data Store Memory : DataStoreMemory  DataStoreName=x0  InitialValue=zeros(1,nS)  ShowAdditionalParam=off  OutDataTypeStr=double
  Data Store Read : DataStoreRead  DataStoreName=x0
  If : If  IfExpression=u1 < nOffset  ShowElse=off
  If Action : Subsystem  TreatAsAtomicUnit=on
  Sum1 : Sum  Inputs=+-|  SaturateOnIntegerOverflow=on  InputSameDT=on  OutDataTypeStr=Inherit: Same as first input
  Switch : Switch  Threshold=nOffset  SaturateOnIntegerOverflow=on  InputSameDT=on
  typeConv : DataTypeConversion  OutDataTypeStr=double  RndMeth=Round  SaturateOnIntegerOverflow=on
  Out1 : Outport
  wires:
  Switch/1 -> Out1/1
  Sum1/1 -> Switch/1
  Data Store Read/1 -> Sum1/2
  In1/1 -> If Action/1(In1), Sum1/1
  Constant/1 -> Switch/3
  Counter/1 -> typeConv/1
  If/1 -> If Action/Action
  typeConv/1 -> Switch/2, If/1

== system HybridControllerD2D2/model/simPC HC/SubSystem0 ==
  In : Inport
  Compare To Constant : simulink/Logic and Bit Operations/Compare To Constant  relop=<  const=0  OutDataTypeStr=boolean
  Detect Fall Nonpositive : simulink/Logic and Bit Operations/Detect Fall Nonpositive  vinit=0  OutDataTypeStr=uint8
      settings: SourceProductName=Simulink  SourceProductBaseCode=SL
  Detect Rise Positive : simulink/Logic and Bit Operations/Detect Rise Positive  vinit=0  OutDataTypeStr=uint8
  If Action Subsystem0 : Subsystem  TreatAsAtomicUnit=on
  If Action Subsystem1 : Subsystem  TreatAsAtomicUnit=on
  If0 : If  IfExpression=u1 == 1  ShowElse=off
  If1 : If  IfExpression=u1 == 1  ShowElse=off
  Mux1 : Mux  Inputs=3
  Stop Simulation : Stop
  typeConv : DataTypeConversion  OutDataTypeStr=int32  RndMeth=Round  SaturateOnIntegerOverflow=on
  Out : Outport
  tag scope: flags=global
  wires:
  Detect Rise Positive/1 -> If0/1, typeConv/1
  Detect Fall Nonpositive/1 -> If1/1
  If1/1 -> If Action Subsystem1/Action
  If0/1 -> If Action Subsystem0/Action
  typeConv/1 -> Out/1
  Mux1/1 -> [flags]
  [sPC] -> Mux1/2
  [atT] -> Mux1/3
  In/1 -> Detect Rise Positive/1, Detect Fall Nonpositive/1, Compare To Constant/1, Mux1/1
  Compare To Constant/1 -> Stop Simulation/1

== system HybridControllerD2D2/model/simPC HC/SubSystem1 ==
  measDsp : Inport
  measFrc : Inport  Port=2
  Constant : Constant  Value=iDelay
  For Each Subsystem : Subsystem  TreatAsAtomicUnit=on
  Gain4 : Gain  SaturateOnIntegerOverflow=on  OutDataTypeStr=Inherit: Same as input  ParamDataTypeStr=Inherit: Same as input
  Mux : Mux  Inputs=2
  SubSystem2 : Subsystem  TreatAsAtomicUnit=on
  Subsystem2 : Subsystem
  measSig : Outport
  tag scope: measDsp=global, measFrc=global
  wires:
  Subsystem2/1(trig) -> SubSystem2/Trigger
  [counter] -> Subsystem2/1(i), For Each Subsystem/1(i)
  Gain4/1 -> measSig/1
  Constant/1 -> For Each Subsystem/2(iDelay)
  measDsp/1 -> [measDsp], For Each Subsystem/3(measDsp)
  measFrc/1 -> For Each Subsystem/4(measFrc), [measFrc]
  For Each Subsystem/1(measDspOut) -> Mux/1
  For Each Subsystem/2(measFrcOut) -> Mux/2
  Mux/1 -> Gain4/1

== system HybridControllerD2D2/model/simPC HC/Subsystem ==
  I : Inport  PortDimensions=nDOF
  Dummy Aug : Mux  Inputs=[nDOF 1]
  Dummy Zero : Constant  Value=0  OutDataTypeStr=double  SampleTime=-1
  O : Outport  PortDimensions=nDOF+1
  tag scope: targSig=global
  wires:
  Dummy Zero/1 -> Dummy Aug/2
  I/1 -> Dummy Aug/1, [targSig]
  Dummy Aug/1 -> O/1

== system HybridControllerD2D2/model/simPC HC/Subsystem1 ==
  In : Inport  PortDimensions=nDOF+1
  Dummy Trn : Demux  Outputs=[nDOF 1]
  Terminator3 : Terminator
  Out : Outport  PortDimensions=nDOF
  tag scope: comSigDot=global
  wires:
  Dummy Trn/2 -> Terminator3/1
  Dummy Trn/1 -> Out/1, [comSigDot]
  In/1 -> Dummy Trn/1

== system HybridControllerD2D2/model/simPC HC/Subsystem2 ==
  In : Inport  PortDimensions=nDOF+1
  Dummy Trn : Demux  Outputs=[nDOF 1]
  Terminator3 : Terminator
  Out : Outport  PortDimensions=nDOF
  tag scope: comSig=global
  wires:
  Dummy Trn/2 -> Terminator3/1
  Dummy Trn/1 -> Out/1, [comSig]
  In/1 -> Dummy Trn/1

== system HybridControllerD2D2/model/simPC HC/Subsystem3 ==
  In : Inport  PortDimensions=nDOF+1
  Dummy Trn : Demux  Outputs=[nDOF 1]
  Terminator3 : Terminator
  Out : Outport  PortDimensions=nDOF
  tag scope: comSigDotDot=global
  wires:
  Dummy Trn/2 -> Terminator3/1
  Dummy Trn/1 -> Out/1, [comSigDotDot]
  In/1 -> Dummy Trn/1

== system HybridControllerD2D2/model/simPC HC/Subsystem4 ==
  BusCreator1 : BusCreator  Inputs=3
  Scope1 : Scope
  Scope2 : Scope
  Scope4 : Scope
  Terminator : Terminator
  Terminator1 : Terminator
  wires:
  [targSig] -> BusCreator1/1
  [comSig] -> BusCreator1/2
  [flags] -> Scope4/1
  [measDsp] -> BusCreator1/3
  BusCreator1/1 -> Scope1/1
  [state] -> Scope2/1
  [counter] -> Terminator/1
  [measFrc] -> Terminator1/1

== system HybridControllerD2D2/model/ActuatorPayloadMdl/dynamic long channel #1/actuator//valve model ==
  note: Note: "1" and "2" denote actuator
      | cylinders on either side of the
      | actuator piston.  With positive
      | valve drive, oil is ported into
      | cylinder 1, resulting in positive
      | displacement.
  note: Auxiliary diagnostic output vector:
      | 1:   valve opening
      | 2:   C1 pressure
      | 3:   C2 pressure
      | 4:   delta pressure
      | 5:   force
      | 6:   velocity
      | 7:   C1 flow
      | 8:   C2 flow
      | 9:   total flow
      | 10: kinematic flow
      | 11: compressibility flow
      | 12: leakage flow
  note: Parameter vector:
      | 1:   oil bulk modulus (force/displ^2)
      | 2:   servovalve delay (sec)
      | 3:   servovalve overlap
      | 4:   rated pressure (force/displ^2)
      | 5:   rated flow at rated pressure (displ^3/sec)
      | 6:   nominal flow at rated pressure (displ^3/sec)
      | 7:   actuator piston area 1 (displ^2)
      | 8:   actuator piston area 2 (displ^2)
      | 9:   actuator usable stroke 1 (displ)
      | 10: actuator usable stroke 2 (displ)
      | 11: actuator end cushion length 1 (displ)
      | 12: actuator end cushion length 2 (displ)
      | 13: actuator parasitic damping factor
      | 14: cross-chamber leakage factor (flow/press)
      | 15: ratio port openings according to area
      | 16: sample period (sec)
      |
      | Conversion factors used for converting
      | signals from external (user) to internal
      | (canonical) units:
      |
      | 17: displacement
      | 18: velocity
      | 19: force
      | 20: pressure
      | 21: flow
  cmd : Inport
  displ : Inport  Port=2
  veloc : Inport  Port=3
  spl press : Inport  Port=4
  rtn press : Inport  Port=5
  abs : Abs  SaturateOnIntegerOverflow=on
  actuator : S-Function  FunctionName=actuator  Parameters=actParamsB  SFunctionDeploymentMode=off  EnableBusSupport=off
  total flow sel : Selector  InputPortWidth=12  IndexOptions=Index vector (dialog)  Indices=9  OutputSizes=1
  force : Outport
  flow : Outport  Port=2
  wires:
  veloc/1 -> actuator/3
  displ/1 -> actuator/2
  actuator/1 -> force/1
  cmd/1 -> actuator/1
  rtn press/1 -> actuator/5
  spl press/1 -> actuator/4
  total flow sel/1 -> abs/1
  actuator/2 -> total flow sel/1
  abs/1 -> flow/1

== system HybridControllerD2D2/model/ActuatorPayloadMdl/dynamic long channel #1/payload ==
  force : Inport
  Sum : Sum  Inputs=+----  SaturateOnIntegerOverflow=on  InputSameDT=on  OutDataTypeStr=Inherit: Same as first input
  damper : Gain  Gain=damperB*damperCanon  SaturateOnIntegerOverflow=on  OutDataTypeStr=Inherit: Same as input  ParamDataTypeStr=Inherit: Same as input
  div : Product  Inputs=*/  SaturateOnIntegerOverflow=on  InputSameDT=on  OutDataTypeStr=Inherit: Same as first input
  double integrator : Subsystem
  friction : Subsystem  mask{friction=frictionB*forceCanon, yieldDispl=yieldDisplB*lengthCanon, hysteresis=0}
      mask prompts: friction "Sliding friction"; yieldDispl "Equiv. yield displacement (in)"; hysteresis "Hysteresis constant"
  mass : Constant  Value=massB*massCanon
  static force : Constant  Value=staticForceB*forceCanon
  term1 : Terminator
  unit dly : UnitDelay  SampleTime=-1  HasFrameUpgradeWarning=on
  unit dly1 : UnitDelay  SampleTime=-1  HasFrameUpgradeWarning=on
  veloc units : Gain  Gain=1/velocCanon  SaturateOnIntegerOverflow=on  OutDataTypeStr=Inherit: Same as input  ParamDataTypeStr=Inherit: Same as input
  displ : Outport
  veloc : Outport  Port=2
  tag scope: ch3a=global
  wires:
  friction/1(force) -> Sum/2  "friction force"
  veloc units/1 -> veloc/1
  Sum/1 -> div/1  "inertial force"
  force/1 -> Sum/1  "total force"
  mass/1 -> div/2
  double integrator/3(acc) -> term1/1
  div/1 -> double integrator/1(accel)
  double integrator/1(displ) -> displ/1, unit dly/1
  double integrator/2(veloc) -> veloc units/1, friction/1(veloc), unit dly1/1
  static force/1 -> Sum/5  "static force"
  damper/1 -> Sum/4  "damper force"
  unit dly1/1 -> damper/1
  [ch3b] -> Sum/3  "spring force"
  unit dly/1 -> [ch3a]
